simulink model "ex_kalman11"  (R2017a)
settings: Solver=FixedStepDiscrete  StartTime=0.0  StopTime=309  RelTol=1e-3  EnableMultiTasking=on
InitFcn:
  | load position.mat;
  | [R,C]=size(position);
  | FRAME_SIZE = 5;
  | idx=(1:FRAME_SIZE:C)';
  | LEN = length(idx);
  | t=(1:LEN)'-1;
undefined symbols (not defined in the file or in its folder): position
settings Model: SimulationMode=accelerator  Creator=The MathWorks, Inc.  LastModifiedBy=Pablo Diaz
settings DataIOCC: LimitDataPoints=on  SaveFormat=Array
settings OptimizationCC: ExpressionDepthLimit=2147483647  LifeSpan=inf
settings DebuggingCC: UnderspecifiedInitializationDetection=Classic  MergeDetectMultiDrivingBlocksExec=none  SolverPrmCheckMsg=warning  FcnCallInpInsideContextMsg=warning  StateNameClashWarn=warning  SFUnexpectedBacktrackingDiag=warning  SFNoUnconditionalDefaultTransitionDiag=warning  SFExecutionAtInitializationDiag=none
settings HardwareCC: ProdBitPerPointer=32  ProdBitPerSizeT=32  ProdBitPerPtrDiffT=32  ProdLargestAtomicFloat=None  ProdIntDivRoundTo=Undefined  ProdEndianess=Unspecified  ProdWordSize=32  ProdHWDeviceType=32-bit Generic
settings ModelReferenceCC: PropagateSignalLabelsOutOfModel=off
settings SFSimCC: SimParseCustomCode=off
settings GRTTargetCC: TargetLangStandard=C89/C90 (ANSI)  GeneratePreprocessorConditionals=Disable all  CombineOutputUpdateFcns=off  GRTInterface=on
settings ConfigComp: CovMetricSettings=dw  CovHtmlReporting=on  CovSaveCumulativeToWorkspaceVar=on  CovSaveSingleToWorkspaceVar=on  CovExternalEMLEnable=off

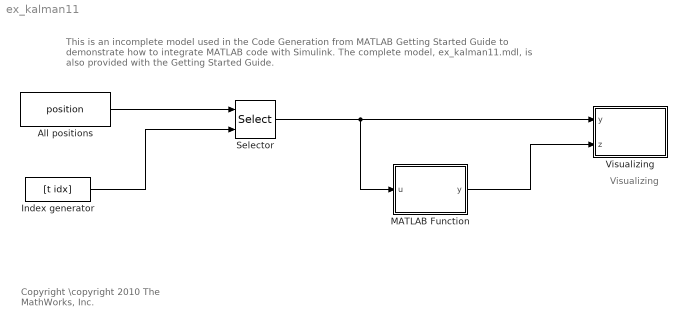
== system ex_kalman11 ==
  note: Visualizing
  note: This is an incomplete model used in the Code Generation from MATLAB Getting Started Guide to demonstrate how to integrate MATLAB code
      | with Simulink.  The complete model,  ex_kalman11.mdl, is also provided with the Getting Started Guide.
  note: Copyright \copyright 2010 The MathWorks, Inc.
  All positions : Constant  Value=position
  Index generator : FromWorkspace  VariableName=[t idx]  SampleTime=1  Interpolate=off  OutputAfterFinalValue=Holding final value
  MATLAB Function : MATLAB Function  TreatAsAtomicUnit=on
  Selector : Selector  NumberOfDimensions=2  InputPortWidth=2  IndexOptions=Select all,Index vector (port)  Indices=[1 3],2  OutputSizes=1,1
  Visualizing : MATLAB Function  TreatAsAtomicUnit=on
  wires:
  All positions/1 -> Selector/1
  Index generator/1 -> Selector/2
  Selector/1 -> MATLAB Function/1(u), Visualizing/1(y)
  MATLAB Function/1(y) -> Visualizing/2(z)

== matlab function ex_kalman11/Visualizing ==
  data: y input; z input
function plot_me(y,z)
%#codegen

coder.extrinsic('figure','hold','plot_trajectory');
persistent h
if isempty(h)
  h=figure;
  hold;
end
plot_trajectory(y,z);
end

== matlab function ex_kalman11/MATLAB Function ==
  data: u input; y output
function y = kalman(u)
%#codegen

y = ex_kalman03(u);
